simulink model "MagnetControlredo"  (Simulink 8.9)
settings: Solver=ode3  StartTime=0.0  StopTime=inf  FixedStep=0.001  RelTol=1e-3  EnableMultiTasking=on
libraries: slrtlib x1, xpcquanserlib x1
settings Model: Creator=Ninad  LastModifiedBy=mishi  SimulationMode=external
settings SolverCC: EnableConcurrentExecution=on
settings OptimizationCC: BlockReduction=off  OptimizeBlockIOStorage=off  BufferReuse=off  GlobalBufferReuse=off  ExpressionFolding=off  ExpressionDepthLimit=2147483647  LocalBlockOutputs=off
settings DebuggingCC: SolverPrmCheckMsg=warning
settings HardwareCC: ProdIntDivRoundTo=Zero  ProdEndianess=LittleEndian  ProdLongLongMode=on  ProdHWDeviceType=Generic->32-bit x86 compatible
settings RTWCC: SystemTargetFile=slrt.tlc  TemplateMakefile=slrt_default_tmf  Description=Simulink Real-Time  CodeExecutionProfiling=on  RTWCompilerOptimization=on
settings SimulinkRealTimeCC: GeneratePreprocessorConditionals=Disable all
settings ConfigComp: CovSFcnEnable=off

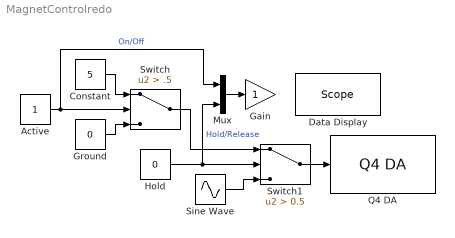
== system MagnetControlredo ==
  Active : Constant
  Constant : Constant  Value=5
  Data Display : slrtlib/Displays and Logging/Scope   scopeno=1  scopetype=Target  autostart=on  viewmode=Numerical  formatstr="'Setpoint        %1d,Motor Position  %1d'"  grid=on  ylimits=[0,170]  nosamples=200  noprepostsamples=0  interleave=10  triggermode=FreeRun  triggersignal=1  trigsignalfromport=off  triggerlevel=0.0  triggerslope=Either  triggerscope=1  triggersample=0  filename=data.dat  mode=Lazy  writesize=512  autorestart=off  dynamicfilemode=off  maxwritefilesize=512*1024^2
  Gain : Gain
  Ground : Constant  Value=0
  Hold : Constant  Value=0
  Mux : Mux  Inputs=2
  "Q4 DA " : xpcquanserlib/D//A/Q4 DA   channel=[2]  range=[-5]  simul=off  reset=[1]  initValue=[0]  sampleTime=.001  slot=-1
      settings: SourceProductName=Simulink Real-Time  SourceProductBaseCode=XP
  Sine Wave : Sin  Amplitude=5  Frequency=2513.27412  Phase=3.14  SampleTime=0
  Switch : Switch  Criteria=u2 > Threshold  Threshold=.5
  Switch1 : Switch  Criteria=u2 > Threshold  Threshold=0.5
  wires:
  Switch1/1 -> "Q4 DA "/1
  Active/1 -> Mux/1, Switch/2  "On/Off"
  Switch/1 -> Switch1/1
  Ground/1 -> Switch/3
  Constant/1 -> Switch/1
  Hold/1 -> Switch1/2, Mux/2  "Hold/Release"
  Mux/1 -> Gain/1
  Sine Wave/1 -> Switch1/3
